simulink model "ards_model"  (R2020b)
settings: Solver=VariableStepAuto  StartTime=0.0  StopTime=480  MaxStep=0.2  RelTol=1e-3
model workspace: external: MAT-File model_workspace.mat (data not in the file)
values from neighbouring files (symbols this model uses):
  C_a_CO2_0 = 0.54    [model_workspace.mat]
  C_a_O2_0 = 0.1974    [model_workspace.mat]
  C_v_CO2_0 = 0.72    [model_workspace.mat]
  C_v_O2_0 = 0.13    [model_workspace.mat]
  moving_average_period = 5    [model_workspace.mat]
  P_ap_0 = 15    [model_workspace.mat]
  P_as_0 = 105.55    [model_workspace.mat]
  P_default = [105.55 4 15 6]    [model_workspace.mat]
  P_vs_0 = 4    [model_workspace.mat]
  Q_0 = 4.8    [model_workspace.mat]
undefined symbols (not defined in the file or in its folder): cRS, Pinsp, VT
libraries: pid_lib x1
(part 2 of 3)

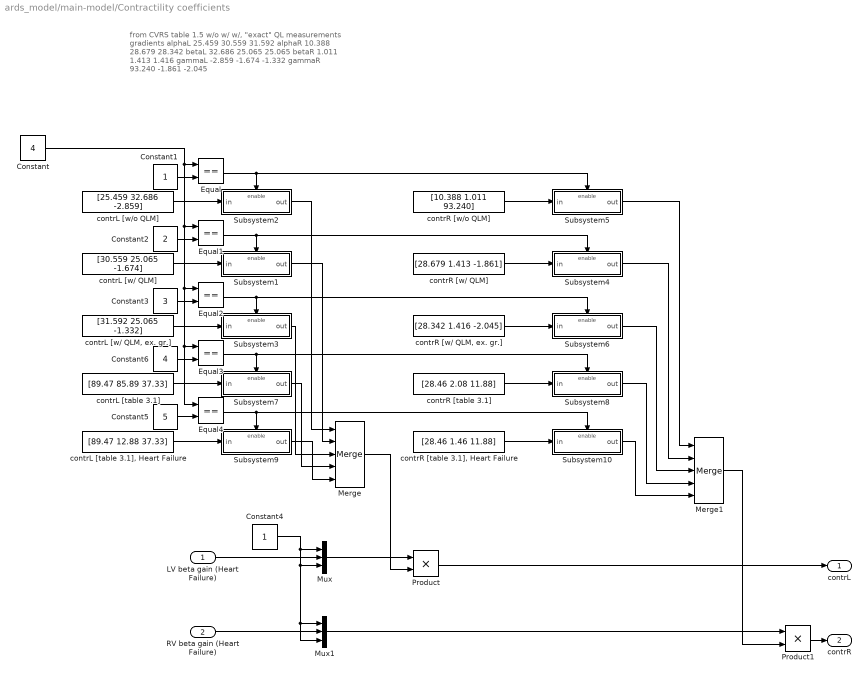
== system ards_model/main-model/Contractility coefficients ==
  note: from CVRS table 1.5
      | w/o w/ w/, "exact"
      | QL measurements gradients
      |
      | alphaL 25.459 30.559 31.592
      | alphaR 10.388 28.679 28.342
      | betaL 32.686 25.065 25.065
      | betaR 1.011 1.413 1.416
      | gammaL -2.859 -1.674 -1.332
      | gammaR 93.240 -1.861 -2.045
  LV beta gain (Heart Failure) : Inport
  RV beta gain (Heart Failure) : Inport  Port=2
  Constant : Constant  Value=4
  Constant1 : Constant
  Constant2 : Constant  Value=2
  Constant3 : Constant  Value=3
  Constant4 : Constant
  Constant5 : Constant  Value=5
  Constant6 : Constant  Value=4
  Equal{,1..4} (5 alike) : RelationalOperator  Operator===  OutDataTypeStr=boolean  RndMeth=Simplest
  Merge : Merge  Inputs=5
  Merge1 : Merge  Inputs=5
  Mux : Mux  Inputs=3
  Mux1 : Mux  Inputs=3
  Product : Product
  Product1 : Product
  Subsystem1 : Subsystem
  Subsystem10 : Subsystem
  Subsystem2 : Subsystem
  Subsystem3 : Subsystem
  Subsystem4 : Subsystem
  Subsystem5 : Subsystem
  Subsystem6 : Subsystem
  Subsystem7 : Subsystem
  Subsystem8 : Subsystem
  Subsystem9 : Subsystem
  contrL [table 3.1] : Constant  Value=[89.47 85.89 37.33]
  "contrL [table 3.1], Heart Failure" : Constant  Value=[89.47 12.88 37.33]
  "contrL [w/ QLM, ex. gr.]" : Constant  Value=[31.592 25.065 -1.332]
  contrL [w/ QLM] : Constant  Value=[30.559 25.065 -1.674]
  contrL [w/o QLM] : Constant  Value=[25.459 32.686 -2.859]
  contrR [table 3.1] : Constant  Value=[28.46 2.08 11.88]
  "contrR [table 3.1], Heart Failure" : Constant  Value=[28.46 1.46 11.88]
  "contrR [w/ QLM, ex. gr.]" : Constant  Value=[28.342 1.416 -2.045]
  contrR [w/ QLM] : Constant  Value=[28.679 1.413 -1.861]
  contrR [w/o QLM] : Constant  Value=[10.388 1.011 93.240]
  contrL : Outport  OutDataTypeStr=double  PortDimensions=3
  contrR : Outport  Port=2  OutDataTypeStr=double  PortDimensions=3
  wires:
  LV beta gain (Heart Failure)/1 -> Mux/2
  RV beta gain (Heart Failure)/1 -> Mux1/2
  Constant/1 -> Equal4/1, Equal3/1, Equal2/1, Equal1/1, Equal/1
  Constant1/1 -> Equal/2
  contrL [w/o QLM]/1 -> Subsystem2/1(in)
  contrL [w/ QLM]/1 -> Subsystem1/1(in)
  "contrL [w/ QLM, ex. gr.]"/1 -> Subsystem3/1(in)
  Equal/1 -> Subsystem5/Enable, Subsystem2/Enable
  Equal1/1 -> Subsystem4/Enable, Subsystem1/Enable
  Constant2/1 -> Equal1/2
  Equal2/1 -> Subsystem6/Enable, Subsystem3/Enable
  Constant3/1 -> Equal2/2
  Subsystem1/1(out) -> Merge/2
  Subsystem2/1(out) -> Merge/1
  Subsystem3/1(out) -> Merge/3
  contrR [w/o QLM]/1 -> Subsystem5/1(in)
  contrR [w/ QLM]/1 -> Subsystem4/1(in)
  "contrR [w/ QLM, ex. gr.]"/1 -> Subsystem6/1(in)
  Subsystem5/1(out) -> Merge1/1
  Subsystem4/1(out) -> Merge1/2
  Subsystem6/1(out) -> Merge1/3
  Constant4/1 -> Mux1/1, Mux1/3, Mux/3, Mux/1
  Mux/1 -> Product/1
  Merge/1 -> Product/2
  Mux1/1 -> Product1/1
  Merge1/1 -> Product1/2
  Product/1 -> contrL/1
  Product1/1 -> contrR/1
  contrL [table 3.1]/1 -> Subsystem7/1(in)
  Constant6/1 -> Equal3/2
  Equal3/1 -> Subsystem8/Enable, Subsystem7/Enable
  Subsystem7/1(out) -> Merge/4
  Subsystem8/1(out) -> Merge1/4
  contrR [table 3.1]/1 -> Subsystem8/1(in)
  "contrR [table 3.1], Heart Failure"/1 -> Subsystem10/1(in)
  Subsystem10/1(out) -> Merge1/5
  Subsystem9/1(out) -> Merge/5
  Equal4/1 -> Subsystem9/Enable, Subsystem10/Enable
  Constant5/1 -> Equal4/2
  "contrL [table 3.1], Heart Failure"/1 -> Subsystem9/1(in)

== system ards_model/main-model/Deadspace by PBW ==
  Weight : Inport  Unit=kg
  Constant1 : Constant  Value=0.0026
  Product2 : Product
  VD : Outport  Unit=L
  wires:
  Constant1/1 -> Product2/2
  Product2/1 -> VD/1  "VD"
  Weight/1 -> Product2/1  "PBW"

== system ards_model/main-model/Initial contractility ==
  H0 : Inport  Unit=1/min
  In3 : Inport  Port=2  OutDataTypeStr=double  PortDimensions=3
  In2 : Inport  Port=3  OutDataTypeStr=double  PortDimensions=3
  Demux : Demux  Outputs=2
  Demux1 : Demux  Outputs=2
  Product : Product  Inputs=*/*
  Product1 : Product  Inputs=*/*
  Selector : Selector  InputPortWidth=3  IndexOptions=Index vector (dialog)  Indices=[1 2]  OutputSizes=1
  Selector1 : Selector  InputPortWidth=3  IndexOptions=Index vector (dialog)  Indices=[1 2]  OutputSizes=1
  SL;0 : Outport  Unit=mmHg
  SR;0 : Outport  Port=2  Unit=mmHg
  wires:
  Product1/1 -> SL;0/1  "SL;0"
  Demux1/2 -> Product/3  "betaR"
  Product/1 -> SR;0/1  "SR;0"
  Demux1/1 -> Product/2  "alphaR"
  Selector/1 -> Demux/1
  Demux/1 -> Product1/2  "alphaL"
  H0/1 -> Product1/1, Product/1  "H0"
  In3/1 -> Selector/1  "contrL"
  Demux/2 -> Product1/3  "betaL"
  In2/1 -> Selector1/1  "contrR"
  Selector1/1 -> Demux1/1

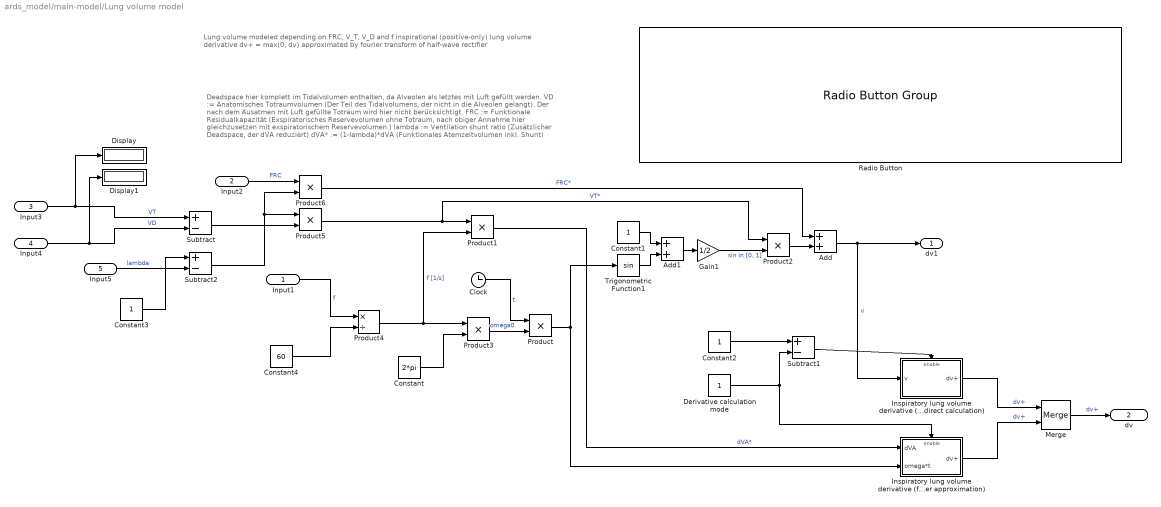
== system ards_model/main-model/Lung volume model ==
  note: Deadspace hier komplett im Tidalvolumen enthalten, da Alveolen als letztes mit Luft gefüllt werden.
      |
      | VD := Anatomisches Totraumvolumen (Der Teil des Tidalvolumens, der nicht in die Alveolen gelangt).
      | 	Der nach dem Ausatmen mit Luft gefüllte Totraum wird hier nicht berücksichtigt.
      | FRC := Funktionale Residualkapazität (Exspiratorisches Reservevolumen ohne Totraum,
      | 	nach obiger Annahme hier gleichzusetzen mit exspiratorischem Reservevolumen.)
      | lambda := Ventilation shunt ratio (Zusätzlicher Deadspace, der dVA reduziert)
      | dVA* := (1-lambda)*dVA (Funktionales Atemzeitvolumen inkl. Shunt)
  note: Lung volume modeled depending on FRC, V_T, V_D and f
      |
      | inspirational (positive-only) lung volume derivative dv+ = max(0, dv) approximated by fourier transform of half-wave rectifier
  Input1 : Inport  Unit=1/min
  Input2 : Inport  Port=2  Unit=L
  Input3 : Inport  Port=3  Unit=L
  Input4 : Inport  Port=4  Unit=L
  Input5 : Inport  Port=5  OutMin=0  OutMax=1  Unit=1
  Add : Sum
  Add1 : Sum
  Clock : Clock
  Constant : Constant  Value=2*pi
  Constant1 : Constant
  Constant2 : Constant
  Constant3 : Constant
  Constant4 : Constant  Value=60
  Derivative calculation mode : Constant
  Display : Display
  Display1 : Display
  Gain1 : Gain  Gain=1/2
  Inspiratory lung volume derivative (direct calculation) : Subsystem
  Inspiratory lung volume derivative (fourier approximation) : Subsystem
  Merge : Merge
  Product{,1..3,5..6} (6 alike) : Product
  Product4 : Product  Inputs=*/
  Radio Button : RadioButtonGroup  SelectedLabel=Fourier approximation (continuous)  ButtonGroupName=Select mode
      settings: Values={{'Direct calculation (with discontinuities)', 'Fourier approximation (continuous)'}, [0 1]}
  Subtract : Sum  Inputs=+-
  Subtract1 : Sum  Inputs=+-
  Subtract2 : Sum  Inputs=+-
  Trigonometric Function1 : Trigonometry
  dv1 : Outport  Unit=L
  dv : Outport  Port=2  Unit=L/s
  wires:
  Product3/1 -> Product/2  "omega0"
  Product4/1 -> Product3/1, Product1/2  "f [1/s]"
  Clock/1 -> Product/1  "t"
  Trigonometric Function1/1 -> Add1/2
  Product2/1 -> Add/2
  Product6/1 -> Add/1  "FRC*"
  Add/1 -> Inspiratory lung volume derivative (direct calculation)/1(v), dv1/1  "v"
  Add1/1 -> Gain1/1
  Constant1/1 -> Add1/1
  Input3/1 -> Display/1, Subtract/1  "VT"
  Input4/1 -> Subtract/2, Display1/1  "VD"
  Constant/1 -> Product3/2
  Product/1 -> Inspiratory lung volume derivative (fourier approximation)/2(omega*t), Trigonometric Function1/1
  Constant4/1 -> Product4/2
  Input1/1 -> Product4/1  "f"
  Gain1/1 -> Product2/2  "sin in [0, 1]"
  Product5/1 -> Product1/1, Product2/1  "VT*"
  Product1/1 -> Inspiratory lung volume derivative (fourier approximation)/1(dVA)  "dVA*"
  Inspiratory lung volume derivative (fourier approximation)/1(dv+) -> Merge/2  "dv+"
  Constant2/1 -> Subtract1/1
  Derivative calculation mode/1 -> Subtract1/2, Inspiratory lung volume derivative (fourier approximation)/Enable
  Inspiratory lung volume derivative (direct calculation)/1(dv+) -> Merge/1  "dv+"
  Merge/1 -> dv/1  "dv+"
  Subtract1/1 -> Inspiratory lung volume derivative (direct calculation)/Enable
  Input5/1 -> Subtract2/2  "lambda"
  Constant3/1 -> Subtract2/1
  Subtract/1 -> Product5/2
  Subtract2/1 -> Product6/2, Product5/1
  Input2/1 -> Product6/1  "FRC"

== system ards_model/main-model/Metabolic Parameters ==
  note: S_T = 50 lit (Fincham-Tehrani)
      | S_T = 13 lit (Tehrani DSS)
  Equivalent gas storage (body tissue) [lit] : Constant  Value=13
  Equivalent gas storage (body tissue) [lit]1 : Constant  Value=50
  Equivalent gas storage (brain) [lit] : Constant  Value=1.1
  "Metabolic rate (CO2, body tissue) [lit/s]" : Constant  Value=0.00287
  "Metabolic rate (CO2, brain) [lit/s]" : Constant  Value=0.0009
  "Metabolic rate (O2, body tissue, positive) [lit/s]" : Constant  Value=0.00352
  "Metabolic rate (O2, brain, positive) [lit/s]" : Constant  Value=0.000925
  Multiply : Gain  Gain=-1
  Multiply1 : Gain  Gain=-1
  Mux : Mux  Inputs=3
  Mux1 : Mux  Inputs=3
  Output : Outport  PortDimensions=3
  Output1 : Outport  Port=2  PortDimensions=3
  wires:
  Equivalent gas storage (body tissue) [lit]1/1 -> Mux/1  "S_T"
  "Metabolic rate (O2, body tissue, positive) [lit/s]"/1 -> Multiply1/1  "-MRT;O2"
  "Metabolic rate (O2, brain, positive) [lit/s]"/1 -> Multiply/1  "-MRB;O2"
  "Metabolic rate (CO2, body tissue) [lit/s]"/1 -> Mux/3  "MRT;CO2"
  Multiply1/1 -> Mux/2  "MRT;O2"
  Multiply/1 -> Mux1/2  "MRB;O2"
  Equivalent gas storage (brain) [lit]/1 -> Mux1/1  "S_B"
  "Metabolic rate (CO2, brain) [lit/s]"/1 -> Mux1/3  "MRB;CO2"
  Mux/1 -> Output/1  "paramsT"
  Mux1/1 -> Output1/1  "paramsB"

== system ards_model/main-model/Predicted Body Weight ==
  note: Predicted body weight
      | Source: Ventilation with lower tidal volumes [...], page 3
  height : Inport  Unit=m
  Input : Inport  Port=2  OutDataTypeStr=boolean
  Add4 : Sum  Inputs=+-
  Constant1 : Constant  Value=1.524
  Constant3 : Constant  Value=0
  Gain : Gain  Gain=91
  IfThenElse : Subsystem
  Max : MinMax  Function=max  Inputs=2
  Subtract1 : Sum
  female : Constant  Value=45.5
  male : Constant  Value=50
  Weight : Outport  Unit=kg
  wires:
  Max/1 -> Gain/1
  Constant1/1 -> Add4/2
  Gain/1 -> Subtract1/1
  Constant3/1 -> Max/2
  height/1 -> Add4/1  "height"
  Subtract1/1 -> Weight/1  "PBW"
  Add4/1 -> Max/1
  female/1 -> IfThenElse/2(then)
  male/1 -> IfThenElse/3(else)
  IfThenElse/1(out) -> Subtract1/2
  Input/1 -> IfThenElse/1(if)  "female"

== system ards_model/main-model/Tissue-Brain fork ratio ==
  note: Tissue-Brain fork ratio
      | Use blood flow rates from [TehraniAbbasi] to calculate fork ratio
  Add : Sum
  Blood flow in body tissue [lit/s] : Constant  Value=0.07083
  Blood flow in brain [lit/s] : Constant  Value=0.0125
  Divide : Product  Inputs=*/
  QT/Qco : Outport  Unit=1
  wires:
  Divide/1 -> QT/Qco/1  "QT/Qs"
  Add/1 -> Divide/2  "qs"
  Blood flow in brain [lit/s]/1 -> Add/2  "qB"
  Blood flow in body tissue [lit/s]/1 -> Divide/1, Add/1  "qT"

== system ards_model/main-model/Total metabolic rate ==
  MRT;O2 : Inport  Unit=L/s
  MRB;O2 : Inport  Port=2  Unit=L/s
  Add : Sum  Inputs=--
  Constant : Constant  Value=60
  Product : Product
  MR_;O2 : Outport  Unit=L/min
  wires:
  Product/1 -> MR_;O2/1  "-MR_;O2"
  Constant/1 -> Product/2
  MRB;O2/1 -> Add/2
  Add/1 -> Product/1
  MRT;O2/1 -> Add/1

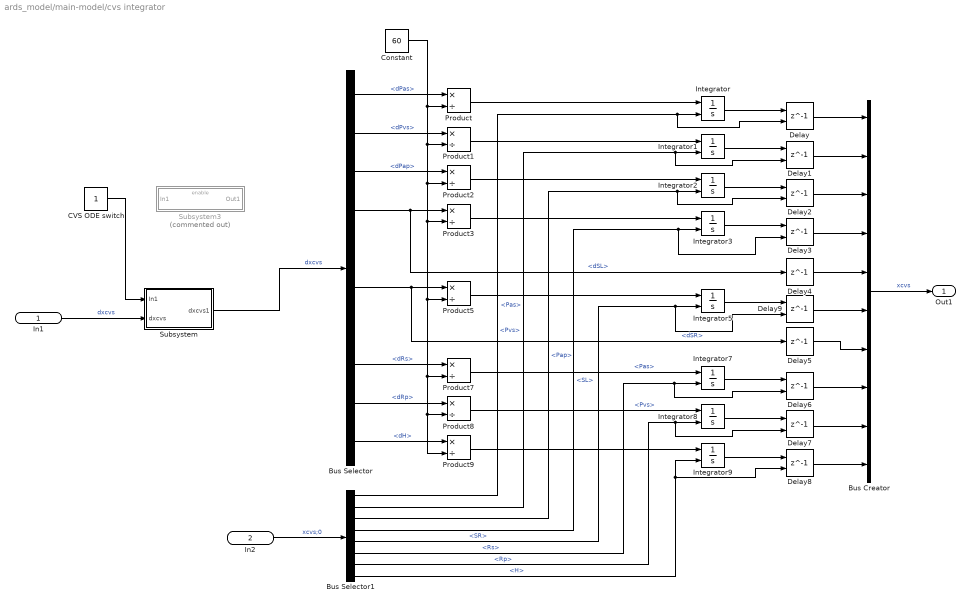
== system ards_model/main-model/cvs integrator ==
  In1 : Inport  OutDataTypeStr=Bus: CardioVascularStateDerivative
  In2 : Inport  Port=2  OutDataTypeStr=Bus: CardioVascularState
  Bus Creator : BusCreator  Inputs=10  OutDataTypeStr=Bus: CardioVascularState
      settings: InheritFromInputs=off
  Bus Selector : BusSelector  OutputSignals=dPas,dPvs,dPap,dSL,dsigmaL,dSR,dsigmaR,dRs,dRp,dH
  Bus Selector1 : BusSelector  OutputSignals=Pas,Pvs,Pap,SL,SR,Rs,Rp,H
  CVS ODE switch : Constant
  Constant : Constant  Value=60
  Delay{,1..3,6..9} (8 alike) : Delay  DelayLength=1  InitialConditionSource=Input port
      settings: InputPortMap=u0,p4
  Delay4 : Delay  DelayLength=1
  Delay5 : Delay  DelayLength=1
  Integrator{,1..3,5,7..9} (8 alike) : Integrator  InitialConditionSource=external
  Product{,1..3,5,7..9} (8 alike) : Product  Inputs=*/
  Subsystem : Subsystem
  Subsystem3 : Subsystem  Commented=on
  Out1 : Outport  OutDataTypeStr=Bus: CardioVascularState
  wires:
  In2/1 -> Bus Selector1/1  "xcvs;0"
  Bus Creator/1 -> Out1/1  "xcvs"
  Bus Selector/1 -> Product/1  "<dPas>"
  Constant/1 -> Product9/2, Product8/2, Product7/2, Product5/2, Product3/2, Product2/2, Product1/2, Product/2
  Product/1 -> Integrator/1
  Product1/1 -> Integrator1/1
  Product2/1 -> Integrator2/1
  Bus Selector/3 -> Product2/1  "<dPap>"
  Bus Selector/2 -> Product1/1  "<dPvs>"
  Product3/1 -> Integrator3/1
  Bus Selector/4 -> Delay4/1, Product3/1  "<dSL>"
  Product9/1 -> Integrator9/1
  Product5/1 -> Integrator5/1
  Bus Selector/6 -> Delay5/1, Product5/1  "<dSR>"
  Bus Selector/8 -> Product7/1  "<dRs>"
  Bus Selector/9 -> Product8/1  "<dRp>"
  Bus Selector/10 -> Product9/1  "<dH>"
  Bus Selector1/1 -> Delay/2, Integrator/2  "<Pas>"
  Bus Selector1/2 -> Delay1/2, Integrator1/2  "<Pvs>"
  Bus Selector1/3 -> Delay2/2, Integrator2/2  "<Pap>"
  Bus Selector1/4 -> Delay3/2, Integrator3/2  "<SL>"
  Bus Selector1/5 -> Delay9/2, Integrator5/2  "<SR>"
  Bus Selector1/6 -> Delay6/2, Integrator7/2  "<Rs>"
  Bus Selector1/7 -> Delay7/2, Integrator8/2  "<Rp>"
  Integrator/1 -> Delay/1
  Integrator1/1 -> Delay1/1
  Integrator2/1 -> Delay2/1
  Integrator3/1 -> Delay3/1
  Delay5/1 -> Bus Creator/7
  Integrator9/1 -> Delay8/1
  Integrator8/1 -> Delay7/1
  Integrator7/1 -> Delay6/1
  Product8/1 -> Integrator8/1  "<Pvs>"
  Product7/1 -> Integrator7/1  "<Pas>"
  Bus Selector1/8 -> Delay8/2, Integrator9/2  "<H>"
  Delay4/1 -> Bus Creator/5
  Delay3/1 -> Bus Creator/4
  Delay2/1 -> Bus Creator/3
  Delay1/1 -> Bus Creator/2
  Delay/1 -> Bus Creator/1
  Delay6/1 -> Bus Creator/8
  Delay7/1 -> Bus Creator/9
  Delay8/1 -> Bus Creator/10
  Integrator5/1 -> Delay9/1
  Delay9/1 -> Bus Creator/6
  Subsystem/1(dxcvs1) -> Bus Selector/1  "dxcvs"
  In1/1 -> Subsystem/2(dxcvs)  "dxcvs"
  CVS ODE switch/1 -> Subsystem/1(In1)

== system ards_model/main-model/cvs_bkst ==
  Input : Inport  OutDataTypeStr=Bus: CardioVascularState
  Input2 : Inport  Port=2  OutDataTypeStr=Bus: CardioVascularState
  Input1 : Inport  Port=3  OutDataTypeStr=Bus: RespiratoryStateExtended
  body surface : Inport  Port=4  Unit=m^2
  CvO1 : Inport  Port=5  Unit=L/min
  Input4 : Inport  Port=6  OutDataTypeStr=double  PortDimensions=3
  Input5 : Inport  Port=7  OutDataTypeStr=double  PortDimensions=3
  Input3 : InportShadow  OutDataTypeStr=Bus: CardioVascularState
  ODEs : Subsystem
  Subsystem : Subsystem
  calculations : Subsystem  ReferencedSubsystem=cvs_calculations
  initial calculations : Subsystem  Commented=on  ReferencedSubsystem=cvs_calculations
  Output : Outport  OutDataTypeStr=Bus: CardioVascularStateDerivative
  Output1 : Outport  Port=2  OutDataTypeStr=Bus: CardioVascularStateExtended
  wires:
  Input/1 -> calculations/1  "xcvs"
  body surface/1 -> initial calculations/2, calculations/2  "surface"
  Input4/1 -> ODEs/3(Input4)  "contrL"
  Input5/1 -> ODEs/4(Input5)  "contrR"
  Input3/1 -> ODEs/5(Input)  "xcvs"
  Input1/1 -> ODEs/6(Input1)  "xrsExt"
  CvO1/1 -> ODEs/7(CvO1)  "-MR_;O2"
  Input2/1 -> initial calculations/1  "xcvs;0"
  calculations/1 -> Subsystem/1(In1)  "xcvsExt"
  ODEs/1(dxcvs [/min]) -> Output/1  "dxcvs"
  calculations/2 -> ODEs/2(c_)
  Subsystem/1(Out1) -> Output1/1, ODEs/1(xcvsExt)

== system ards_model/main-model/rs integrator ==
  In1 : Inport  OutDataTypeStr=Bus: RespiratoryStateDerivative
  In2 : Inport  Port=2  OutDataTypeStr=Bus: RespiratoryState
  Bus Creator1 : BusCreator  Inputs=6  OutDataTypeStr=Bus: RespiratoryState
      settings: InheritFromInputs=off
  Bus Selector1 : BusSelector  OutputSignals=dPaxO2,dPaxCO2,dCvBO2,dCvBCO2,dCvTO2,dCvTCO2
  Bus Selector2 : BusSelector  OutputSignals=PaxO2,PaxCO2,CvBO2,CvBCO2,CvTO2,CvTCO2
  Delay{,1..5} (6 alike) : Delay  DelayLength=1  InitialConditionSource=Input port
      settings: InputPortMap=u0,p4
  Integrator{,1..5} (6 alike) : Integrator  InitialConditionSource=external
  RS ODE switch : Constant
  Subsystem : Subsystem
  Out1 : Outport  OutDataTypeStr=Bus: RespiratoryState
  wires:
  Integrator/1 -> Delay/1
  Bus Selector2/3 -> Integrator2/2, Delay2/2  "<CvBO2>"
  Bus Selector2/6 -> Delay5/2, Integrator5/2  "<CvTCO2>"
  Bus Selector2/1 -> Delay/2, Integrator/2  "<PaxO2>"
  Bus Selector2/2 -> Delay1/2, Integrator1/2  "<PaxCO2>"
  Integrator4/1 -> Delay4/1
  Integrator2/1 -> Delay2/1
  Bus Selector1/4 -> Integrator3/1  "<dCvBCO2>"
  Integrator1/1 -> Delay1/1
  Integrator5/1 -> Delay5/1
  Bus Selector1/3 -> Integrator2/1  "<dCvBO2>"
  Bus Selector2/4 -> Delay3/2, Integrator3/2  "<CvBCO2>"
  Delay1/1 -> Bus Creator1/2
  Bus Selector1/5 -> Integrator4/1  "<dCvTO2>"
  Delay4/1 -> Bus Creator1/5
  Delay2/1 -> Bus Creator1/3
  Bus Selector2/5 -> Delay4/2, Integrator4/2  "<CvTO2>"
  Delay5/1 -> Bus Creator1/6
  Integrator3/1 -> Delay3/1
  Delay3/1 -> Bus Creator1/4
  Delay/1 -> Bus Creator1/1
  Bus Selector1/1 -> Integrator/1  "<dPaxO2>"
  Bus Selector1/6 -> Integrator5/1  "<dCvTCO2>"
  Bus Selector1/2 -> Integrator1/1  "<dPaxCO2>"
  Bus Creator1/1 -> Out1/1  "xrs"
  In2/1 -> Bus Selector2/1  "xrs;0"
  Subsystem/1(dxcvs1) -> Bus Selector1/1  "dxrs"
  RS ODE switch/1 -> Subsystem/1(In1)
  In1/1 -> Subsystem/2(dxcvs)  "dxrs"

== system ards_model/main-model/rs_tehrani ==
  Qco7 : Inport  OutDataTypeStr=Bus: RespiratoryState  Unit=liter/minute
  Qco2 : Inport  Port=2  OutDataTypeStr=Bus: RespiratoryState  Unit=liter/minute
  Qco : Inport  Port=3  OutDataTypeStr=Bus: CardioVascularStateExtended  Unit=liter/minute
  v : Inport  Port=4  Unit=L
  dv+ : Inport  Port=5  Unit=liter/second
  Pamb* : Inport  Port=6  Unit=mmHg
  Fi;O2 : Inport  Port=7  Unit=1
  Fi;CO2 : Inport  Port=8  Unit=1
  rho : Inport  Port=9  Unit=1
  QT8 : Inport  Port=10  PortDimensions=3
  QT4 : Inport  Port=11  PortDimensions=3
  QT;0/Qco;0 : Inport  Port=12  Unit=1
  Fi;O1 : InportShadow  Port=7  Unit=1
  ODEs : Subsystem
  calculations : Subsystem  ReferencedSubsystem=tehrani_rs_calculations
  initial calculations : Subsystem  Commented=on  ReferencedSubsystem=tehrani_rs_calculations
  Output : Outport  OutDataTypeStr=Bus: RespiratoryStateDerivative
  Output1 : Outport  Port=2  OutDataTypeStr=Bus: RespiratoryStateExtended
  wires:
  Qco/1 -> initial calculations/2, calculations/2  "xcvsExt"
  Fi;O1/1 -> initial calculations/3, calculations/3  "Fi;O2"
  rho/1 -> initial calculations/4, calculations/4  "rho"
  QT;0/Qco;0/1 -> initial calculations/5, calculations/5  "QT/Qs"
  Qco7/1 -> calculations/1  "xrs"
  Qco2/1 -> initial calculations/1  "xrs0"
  Pamb*/1 -> ODEs/5(Pamb*)  "Pamb"
  v/1 -> ODEs/6(v)  "v"
  dv+/1 -> ODEs/7(dv+)  "dv+"
  Fi;O2/1 -> ODEs/8(Fi;O2)  "Fi;O2"
  Fi;CO2/1 -> ODEs/9(Fi;CO2)  "Fi;CO2"
  calculations/2 -> ODEs/2(inpp*)
  calculations/3 -> ODEs/3(inpB)
  calculations/4 -> ODEs/4(inpT)
  ODEs/1(dxrs) -> Output/1  "dxrs"
  QT8/1 -> ODEs/11(QT1)  "paramsT"
  QT4/1 -> ODEs/10(QT4)  "paramsB"
  calculations/1 -> Output1/1, ODEs/1(xrsExt)  "xrsExt"

== system ards_model/Predicted Body Weight/IfThenElse/Subsystem1 ==
  in : Inport
  Enable : EnablePort
  out : Outport
  wires:
  in/1 -> out/1

== system ards_model/Predicted Body Weight/IfThenElse/Subsystem2 ==
  in : Inport
  Enable : EnablePort
  out : Outport
  wires:
  in/1 -> out/1

== system ards_model/ards_classification/ARDS level score calculation/Subsystem ==
  in : Inport
  Enable : EnablePort
  out : Outport
  wires:
  in/1 -> out/1

== system ards_model/ards_classification/ARDS level score calculation/Subsystem1 ==
  in : Inport
  Enable : EnablePort
  out : Outport
  wires:
  in/1 -> out/1

== system ards_model/ards_classification/ARDS level score calculation/Subsystem2 ==
  in : Inport
  Enable : EnablePort
  out : Outport
  wires:
  in/1 -> out/1

== system ards_model/ards_classification/ARDS level score calculation/Subsystem3 ==
  in : Inport
  Enable : EnablePort
  out : Outport
  wires:
  in/1 -> out/1

== system ards_model/ards_classification/Berlin definition/PEEP bound ==
  PEEP : Inport  Unit=mbar
  Constant : Constant  Value=5
  GreaterThanOrEqual : RelationalOperator  OutDataTypeStr=boolean  RndMeth=Simplest
  Subsystem2 : Subsystem  ReferencedSubsystem=convert_mbar_to_cmh2o
  Out1 : Outport  OutDataTypeStr=boolean
  wires:
  Constant/1 -> GreaterThanOrEqual/2
  Subsystem2/1 -> GreaterThanOrEqual/1  "PEEP [cmH2O]"
  GreaterThanOrEqual/1 -> Out1/1  "ispeep"
  PEEP/1 -> Subsystem2/1

== system ards_model/ards_classification/Berlin definition/ards_level ==
  horowitz : Inport  Unit=mmHg
  Fi;O2 : Inport  Port=2  Unit=1
  altitude : Inport  Port=3  Unit=m
  Pamb : Inport  Port=4  Unit=mmHg
  Input : Inport  Port=5
  AND : Logic  IconShape=distinctive  AllPortsSameDT=off  OutDataTypeStr=boolean
  AND1 : Logic  IconShape=distinctive  AllPortsSameDT=off  OutDataTypeStr=boolean
  AND2 : Logic  IconShape=distinctive  AllPortsSameDT=off  OutDataTypeStr=boolean
  NOT : Logic  Operator=NOT  IconShape=distinctive  AllPortsSameDT=off  OutDataTypeStr=boolean
  NOT1 : Logic  Operator=NOT  IconShape=distinctive  AllPortsSameDT=off  OutDataTypeStr=boolean
  OR : Logic  Operator=OR  IconShape=distinctive  AllPortsSameDT=off  OutDataTypeStr=boolean
  ards_level_string : Subsystem
  ards_level_switch : Subsystem
  Out1 : Outport
  ards : Outport  Port=2
  no : Outport  Port=3
  mild : Outport  Port=4
  moderate : Outport  Port=5
  severe : Outport  Port=6
  wires:
  AND/1 -> ards_level_string/1(In1), severe/1  "severe"
  AND2/1 -> ards_level_string/3(In3), mild/1  "mild"
  AND1/1 -> ards_level_string/2(In2), moderate/1  "moderate"
  horowitz/1 -> ards_level_switch/1(horowitz)
  Pamb/1 -> ards_level_switch/4(Pamb)
  ards_level_string/1(ards_level) -> Out1/1  "level_string"
  NOT/1 -> ards/1  "ards"
  Input/1 -> AND2/2, AND1/2, AND/2, NOT1/1  "ispeep"
  ards_level_switch/1(issevere) -> AND/1  "severe"
  ards_level_switch/2(ismoderate) -> AND1/1  "moderate"
  ards_level_switch/3(ismild) -> AND2/1  "mild"
  OR/1 -> ards_level_string/4(In4), NOT/1, no/1  "no"
  ards_level_switch/4(isno) -> OR/1  "no"
  NOT1/1 -> OR/2
  altitude/1 -> ards_level_switch/3(Pamb1)
  Fi;O2/1 -> ards_level_switch/2(horowitz1)

== system ards_model/ards_classification/LVEF_score/Enabled Subsystem ==
  In1 : Inport
  Enable : EnablePort
  Out1 : Outport
  wires:
  In1/1 -> Out1/1

== system ards_model/ards_classification/LVEF_score/Enabled Subsystem1 ==
  In1 : Inport
  Enable : EnablePort
  Out1 : Outport
  wires:
  In1/1 -> Out1/1

== system ards_model/ards_classification/LVEF_score/Enabled Subsystem2 ==
  In1 : Inport
  Enable : EnablePort
  Out1 : Outport
  wires:
  In1/1 -> Out1/1

== system ards_model/ards_classification/NTproBNP_score/Enabled Subsystem ==
  In1 : Inport
  Enable : EnablePort
  Out1 : Outport
  wires:
  In1/1 -> Out1/1

== system ards_model/ards_classification/NTproBNP_score/Enabled Subsystem1 ==
  In1 : Inport
  Enable : EnablePort
  Out1 : Outport
  wires:
  In1/1 -> Out1/1

== system ards_model/ards_classification/NTproBNP_score/Enabled Subsystem2 ==
  In1 : Inport
  Enable : EnablePort
  Out1 : Outport
  wires:
  In1/1 -> Out1/1

== system ards_model/ards_classification/RHF_risk_level_string/Subsystem ==
  in : Inport
  Enable : EnablePort
  out : Outport
  wires:
  in/1 -> out/1

== system ards_model/ards_classification/RHF_risk_level_string/Subsystem1 ==
  in : Inport
  Enable : EnablePort
  out : Outport
  wires:
  in/1 -> out/1

== system ards_model/ards_classification/RHF_risk_level_string/Subsystem2 ==
  in : Inport
  Enable : EnablePort
  out : Outport
  wires:
  in/1 -> out/1

== system ards_model/ards_classification/RHF_risk_level_string/Subsystem3 ==
  in : Inport
  Enable : EnablePort
  out : Outport
  wires:
  in/1 -> out/1

== system ards_model/ards_classification/eGFR_CKD-EPI/alpha ==
  In1 : Inport
  Constant : Constant
  Enabled Subsystem : Subsystem  TreatAsAtomicUnit=on
  Enabled Subsystem1 : Subsystem  TreatAsAtomicUnit=on
  Equal : RelationalOperator  Operator===  OutDataTypeStr=boolean  RndMeth=Simplest
  Merge : Merge
  NOT : Logic  Operator=NOT  IconShape=distinctive  AllPortsSameDT=off  OutDataTypeStr=boolean
  alphaM : Constant  Value=-0.411
  alphaW : Constant  Value=-0.329
  Out1 : Outport
  wires:
  Merge/1 -> Out1/1
  Enabled Subsystem/1(Out1) -> Merge/1
  NOT/1 -> Enabled Subsystem1/Enable
  alphaM/1 -> Enabled Subsystem1/1(In1)
  alphaW/1 -> Enabled Subsystem/1(In1)
  In1/1 -> Enabled Subsystem/Enable, NOT/1
  Enabled Subsystem1/1(Out1) -> Merge/2
  Constant/1 -> Equal/1

== system ards_model/ards_classification/eGFR_CKD-EPI/kappa ==
  In1 : Inport
  Constant : Constant
  Enabled Subsystem : Subsystem  TreatAsAtomicUnit=on
  Enabled Subsystem1 : Subsystem  TreatAsAtomicUnit=on
  Equal : RelationalOperator  Operator===  OutDataTypeStr=boolean  RndMeth=Simplest
  Merge : Merge
  NOT : Logic  Operator=NOT  IconShape=distinctive  AllPortsSameDT=off  OutDataTypeStr=boolean
  kappaM : Constant  Value=0.9
  kappaW : Constant  Value=0.7
  Out1 : Outport
  wires:
  Enabled Subsystem1/1(Out1) -> Merge/2
  In1/1 -> Enabled Subsystem/Enable, NOT/1
  kappaW/1 -> Enabled Subsystem/1(In1)
  kappaM/1 -> Enabled Subsystem1/1(In1)
  NOT/1 -> Enabled Subsystem1/Enable
  Enabled Subsystem/1(Out1) -> Merge/1
  Merge/1 -> Out1/1
  Constant/1 -> Equal/1

== system ards_model/ards_classification/eGFR_CKD-EPI/sex factor ==
  In1 : Inport
  Constant : Constant
  Enabled Subsystem : Subsystem  TreatAsAtomicUnit=on
  Enabled Subsystem1 : Subsystem  TreatAsAtomicUnit=on
  Equal : RelationalOperator  Operator===  OutDataTypeStr=boolean  RndMeth=Simplest
  M : Constant
  Merge : Merge
  NOT : Logic  Operator=NOT  IconShape=distinctive  AllPortsSameDT=off  OutDataTypeStr=boolean
  W : Constant  Value=1.018
  Out1 : Outport
  wires:
  Enabled Subsystem1/1(Out1) -> Merge/2
  In1/1 -> Enabled Subsystem/Enable, NOT/1
  W/1 -> Enabled Subsystem/1(In1)
  M/1 -> Enabled Subsystem1/1(In1)
  NOT/1 -> Enabled Subsystem1/Enable
  Enabled Subsystem/1(Out1) -> Merge/1
  Merge/1 -> Out1/1
  Constant/1 -> Equal/1

== system ards_model/ards_classification/eGFR_CKD-EPI/skin color factor ==
  In1 : Inport
  B : Constant  Value=1.159
  Constant : Constant
  Enabled Subsystem : Subsystem  TreatAsAtomicUnit=on
  Enabled Subsystem1 : Subsystem  TreatAsAtomicUnit=on
  Equal : RelationalOperator  Operator===  OutDataTypeStr=boolean  RndMeth=Simplest
  Merge : Merge
  NOT : Logic  Operator=NOT  IconShape=distinctive  AllPortsSameDT=off  OutDataTypeStr=boolean
  W : Constant
  Out1 : Outport
  wires:
  Merge/1 -> Out1/1
  Enabled Subsystem/1(Out1) -> Merge/1
  NOT/1 -> Enabled Subsystem1/Enable
  W/1 -> Enabled Subsystem1/1(In1)
  B/1 -> Enabled Subsystem/1(In1)
  In1/1 -> NOT/1, Enabled Subsystem/Enable
  Enabled Subsystem1/1(Out1) -> Merge/2
  Constant/1 -> Equal/1

== system ards_model/ards_classification/logFon_score/Compliance ==
  <height> : Inport  Unit=m
  <weight> : Inport  Port=2  Unit=kg
  Blood volume estimate : Subsystem  TreatAsAtomicUnit=on
  Body surface estimate : Subsystem  TreatAsAtomicUnit=on
  Initial blood volume distribution : Subsystem  TreatAsAtomicUnit=on
  Mux : Mux
  Selector : Selector  InputPortWidth=4  IndexOptions=Index vector (dialog)  Indices=[1]  OutputSizes=1
  Vessel compliances : Subsystem  TreatAsAtomicUnit=on
  cas : Outport  Unit=L/mmHg
  wires:
  Mux/1 -> Selector/1  "c_"
  Vessel compliances/1(cas) -> Mux/1  "cas"
  Vessel compliances/4(cvp) -> Mux/4  "cvp"
  Blood volume estimate/1(Vtot) -> Initial blood volume distribution/1(Vtot)  "Vtot"
  Initial blood volume distribution/4(V_as3) -> Vessel compliances/4(In8)  "Vvp;0"
  Vessel compliances/3(cap) -> Mux/3  "cap"
  Initial blood volume distribution/2(V_as1) -> Vessel compliances/2(In6)  "Vvs;0"
  Initial blood volume distribution/1(V_as) -> Vessel compliances/1(In5)  "Vas;0"
  Vessel compliances/2(cvs) -> Mux/2  "cvs"
  Body surface estimate/1(surface) -> Blood volume estimate/1(surface)  "surface"
  Initial blood volume distribution/3(V_as2) -> Vessel compliances/3(In7)  "Vap;0"
  <weight>/1 -> Body surface estimate/2(Weight)
  Selector/1 -> cas/1  "cas"
  <height>/1 -> Body surface estimate/1(height)

== system ards_model/ards_classification/logFon_score/peak Pas ==
  note: MAP = DBP + tau_syst * (SBP - DBP)
      | [Moran et al.: "Calculation of mean arterial pressure during exercise as a function of Heart Rate"]
  <Pas> : Inport
  <H> : Inport  Port=2
  <Vstr> : Inport  Port=3
  cas : Inport  Port=4
  Add : Sum
  Add1 : Sum
  Add2 : Sum  Inputs=+-
  Constant : Constant  Value=40
  Constant1 : Constant
  Divide : Product  Inputs=*/
  Divide1 : Product  Inputs=*/
  Duration of heart cycle : Subsystem  TreatAsAtomicUnit=on  ReferencedSubsystem=cvrs_heart_cycle
  Max : MinMax  Function=max  Inputs=2
  Product : Product
  Product1 : Product
  Subtract : Sum  Inputs=+-
  Pas;diast : Outport
  Pas;syst : Outport  Port=2
  wires:
  Add/1 -> Divide1/2
  Product/1 -> Add1/2
  Constant1/1 -> Subtract/1
  Duration of heart cycle/2 -> Add/2, Divide1/1  "tsyst"
  Divide/1 -> Product1/2, Product/2  "deltaPas"
  Duration of heart cycle/1 -> Add/1  "tdiast"
  Subtract/1 -> Product/1  "taudiast"
  cas/1 -> Divide/2
  Divide1/1 -> Product1/1, Subtract/2  "tausyst"
  <Vstr>/1 -> Divide/1
  Add1/1 -> Pas;syst/1  "Pas;syst"
  <Pas>/1 -> Add2/1, Add1/1
  Max/1 -> Duration of heart cycle/1
  Constant/1 -> Max/2
  <H>/1 -> Max/1
  Product1/1 -> Add2/2
  Add2/1 -> Pas;diast/1  "Pas;diast"

== system ards_model/main-model/Contractility coefficients/Subsystem1 ==
  in : Inport  OutDataTypeStr=double  PortDimensions=3
  Enable : EnablePort
  out : Outport  OutDataTypeStr=double  PortDimensions=3
  wires:
  in/1 -> out/1

== system ards_model/main-model/Contractility coefficients/Subsystem10 ==
  in : Inport  OutDataTypeStr=double  PortDimensions=3
  Enable : EnablePort
  out : Outport  OutDataTypeStr=double  PortDimensions=3
  wires:
  in/1 -> out/1

== system ards_model/main-model/Contractility coefficients/Subsystem2 ==
  in : Inport  OutDataTypeStr=double  PortDimensions=3
  Enable : EnablePort
  out : Outport  OutDataTypeStr=double  PortDimensions=3
  wires:
  in/1 -> out/1

== system ards_model/main-model/Contractility coefficients/Subsystem3 ==
  in : Inport  OutDataTypeStr=double  PortDimensions=3
  Enable : EnablePort
  out : Outport  OutDataTypeStr=double  PortDimensions=3
  wires:
  in/1 -> out/1

== system ards_model/main-model/Contractility coefficients/Subsystem4 ==
  in : Inport  OutDataTypeStr=double  PortDimensions=3
  Enable : EnablePort
  out : Outport  OutDataTypeStr=double  PortDimensions=3
  wires:
  in/1 -> out/1

== system ards_model/main-model/Contractility coefficients/Subsystem5 ==
  in : Inport  OutDataTypeStr=double  PortDimensions=3
  Enable : EnablePort
  out : Outport  OutDataTypeStr=double  PortDimensions=3
  wires:
  in/1 -> out/1

== system ards_model/main-model/Contractility coefficients/Subsystem6 ==
  in : Inport  OutDataTypeStr=double  PortDimensions=3
  Enable : EnablePort
  out : Outport  OutDataTypeStr=double  PortDimensions=3
  wires:
  in/1 -> out/1

== system ards_model/main-model/Contractility coefficients/Subsystem7 ==
  in : Inport  OutDataTypeStr=double  PortDimensions=3
  Enable : EnablePort
  out : Outport  OutDataTypeStr=double  PortDimensions=3
  wires:
  in/1 -> out/1

== system ards_model/main-model/Contractility coefficients/Subsystem8 ==
  in : Inport  OutDataTypeStr=double  PortDimensions=3
  Enable : EnablePort
  out : Outport  OutDataTypeStr=double  PortDimensions=3
  wires:
  in/1 -> out/1

== system ards_model/main-model/Contractility coefficients/Subsystem9 ==
  in : Inport  OutDataTypeStr=double  PortDimensions=3
  Enable : EnablePort
  out : Outport  OutDataTypeStr=double  PortDimensions=3
  wires:
  in/1 -> out/1

== system ards_model/main-model/Lung volume model/Inspiratory lung volume derivative (direct calculation) ==
  v : Inport
  Enable : EnablePort
  Constant3 : Constant  Value=0
  Derivative : Derivative
  Max : MinMax  Function=max  Inputs=2
  dv+ : Outport
  wires:
  Constant3/1 -> Max/2
  v/1 -> Derivative/1
  Max/1 -> dv+/1  "dv+"
  Derivative/1 -> Max/1

== system ards_model/main-model/Lung volume model/Inspiratory lung volume derivative (fourier approximation) ==
  dVA : Inport
  omega*t : Inport  Port=2
  Enable : EnablePort
  Add2 : Sum
  Gain : Gain  Gain=pi
  Half-wave rectifier : Subsystem
  zero-prevention threshold : Constant  Value=0.01
  dv+ : Outport
  wires:
  omega*t/1 -> Half-wave rectifier/2(2pift)
  zero-prevention threshold/1 -> Add2/2
  Half-wave rectifier/1(out) -> Gain/1
  Add2/1 -> dv+/1  "dv+"
  Gain/1 -> Add2/1
  dVA/1 -> Half-wave rectifier/1((d)VA)

== system ards_model/main-model/Predicted Body Weight/IfThenElse ==
  if : Inport  OutDataTypeStr=boolean
  then : Inport  Port=2
  else : Inport  Port=3
  Merge : Merge
  NOT : Logic  Operator=NOT  IconShape=distinctive  AllPortsSameDT=off  OutDataTypeStr=boolean
  Subsystem1 : Subsystem
  Subsystem2 : Subsystem
  out : Outport
  wires:
  then/1 -> Subsystem1/1(in)
  Subsystem2/1(out) -> Merge/2
  if/1 -> NOT/1, Subsystem1/Enable
  else/1 -> Subsystem2/1(in)
  Subsystem1/1(out) -> Merge/1
  NOT/1 -> Subsystem2/Enable
  Merge/1 -> out/1

== system ards_model/main-model/cvs integrator/Subsystem ==
  In1 : Inport
  dxcvs : Inport  Port=2
  Bus Creator1 : BusCreator  Inputs=10  OutDataTypeStr=Bus: CardioVascularStateDerivative
      settings: InheritFromInputs=off
  Bus to Vector : BusToVector
  Demux1 : Demux  Outputs=10
  Product : Product
  dxcvs1 : Outport
  wires:
  Demux1/6 -> Bus Creator1/6
  Demux1/8 -> Bus Creator1/8
  Demux1/7 -> Bus Creator1/7
  Demux1/5 -> Bus Creator1/5
  Product/1 -> Demux1/1
  Bus to Vector/1 -> Product/2
  Demux1/4 -> Bus Creator1/4
  Demux1/9 -> Bus Creator1/9
  Demux1/10 -> Bus Creator1/10
  Demux1/1 -> Bus Creator1/1
  Demux1/2 -> Bus Creator1/2
  Demux1/3 -> Bus Creator1/3
  Bus Creator1/1 -> dxcvs1/1  "dxcvs"
  In1/1 -> Product/1  "a"
  dxcvs/1 -> Bus to Vector/1  "dxcvs"

== system ards_model/main-model/cvs integrator/Subsystem3 ==
  In1 : Inport  OutDataTypeStr=Bus: CardioVascularStateDerivative
  Enable : EnablePort
  Out1 : Outport  OutDataTypeStr=Bus: CardioVascularStateDerivative
  wires:
  In1/1 -> Out1/1

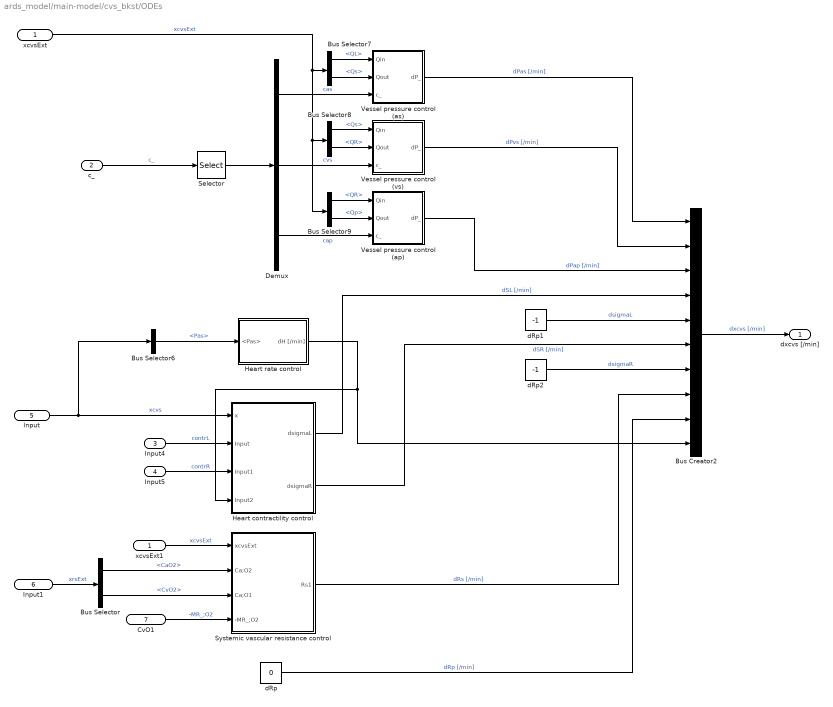
== system ards_model/main-model/cvs_bkst/ODEs ==
  xcvsExt : Inport  OutDataTypeStr=Bus: CardioVascularStateExtended
  c_ : Inport  Port=2  Unit=L/mmHg
  Input4 : Inport  Port=3  OutDataTypeStr=double  PortDimensions=3
  Input5 : Inport  Port=4  OutDataTypeStr=double  PortDimensions=3
  Input : Inport  Port=5  OutDataTypeStr=Bus: CardioVascularState
  Input1 : Inport  Port=6  OutDataTypeStr=Bus: RespiratoryStateExtended
  CvO1 : Inport  Port=7  Unit=L/min
  Bus Creator2 : BusCreator  Inputs=10  OutDataTypeStr=Bus: CardioVascularStateDerivative
  Bus Selector : BusSelector  OutputSignals=CaO2,CvO2
  Bus Selector6 : BusSelector  OutputSignals=Pas
  Bus Selector7 : BusSelector  OutputSignals=QL,Qs
  Bus Selector8 : BusSelector  OutputSignals=Qs,QR
  Bus Selector9 : BusSelector  OutputSignals=QR,Qp
  Demux : Demux  Outputs=3
  Heart contractility control : Subsystem
  Heart rate control : Subsystem
  Selector : Selector  InputPortWidth=4  IndexOptions=Index vector (dialog)  Indices=[1 2 3]  OutputSizes=1
  Systemic vascular resistance control : Subsystem
  Vessel pressure control (ap) : Subsystem
  Vessel pressure control (as) : Subsystem
  Vessel pressure control (vs) : Subsystem
  dRp : Constant  Value=0
  dRp1 : Constant  Value=-1
  dRp2 : Constant  Value=-1
  xcvsExt1 : InportShadow  OutDataTypeStr=Bus: CardioVascularStateExtended
  dxcvs [/min] : Outport  OutDataTypeStr=Bus: CardioVascularStateDerivative
  wires:
  Vessel pressure control (ap)/1(dP_) -> Bus Creator2/3  "dPap [/min]"
  Bus Selector8/1 -> Vessel pressure control (vs)/1(Qin)  "<Qs>"
  Vessel pressure control (vs)/1(dP_) -> Bus Creator2/2  "dPvs [/min]"
  CvO1/1 -> Systemic vascular resistance control/4(-MR_;O2)  "-MR_;O2"
  Demux/2 -> Vessel pressure control (vs)/3(c_)  "cvs"
  Bus Selector9/1 -> Vessel pressure control (ap)/1(Qin)  "<QR>"
  c_/1 -> Selector/1  "c_"
  Heart contractility control/1(dsigmaL) -> Bus Creator2/4  "dSL [/min]"
  Vessel pressure control (as)/1(dP_) -> Bus Creator2/1  "dPas [/min]"
  Demux/1 -> Vessel pressure control (as)/3(c_)  "cas"
  Systemic vascular resistance control/1(Rs1) -> Bus Creator2/8  "dRs [/min]"
  dRp/1 -> Bus Creator2/9  "dRp [/min]"
  xcvsExt/1 -> Bus Selector9/1, Bus Selector8/1, Bus Selector7/1  "xcvsExt"
  dRp2/1 -> Bus Creator2/7  "dsigmaR"
  xcvsExt1/1 -> Systemic vascular resistance control/1(xcvsExt)  "xcvsExt"
  Input/1 -> Heart contractility control/1(x), Bus Selector6/1  "xcvs"
  Input4/1 -> Heart contractility control/2(Input)  "contrL"
  Heart contractility control/2(dsigmaR) -> Bus Creator2/6  "dSR [/min]"
  dRp1/1 -> Bus Creator2/5  "dsigmaL"
  Input5/1 -> Heart contractility control/3(Input1)  "contrR"
  Bus Selector9/2 -> Vessel pressure control (ap)/2(Qout)  "<Qp>"
  Demux/3 -> Vessel pressure control (ap)/3(c_)  "cap"
  Selector/1 -> Demux/1
  Bus Creator2/1 -> dxcvs [/min]/1  "dxcvs [/min]"
  Bus Selector7/2 -> Vessel pressure control (as)/2(Qout)  "<Qs>"
  Bus Selector7/1 -> Vessel pressure control (as)/1(Qin)  "<QL>"
  Bus Selector/1 -> Systemic vascular resistance control/2(Ca;O2)  "<CaO2>"
  Input1/1 -> Bus Selector/1  "xrsExt"
  Bus Selector8/2 -> Vessel pressure control (vs)/2(Qout)  "<QR>"
  Bus Selector/2 -> Systemic vascular resistance control/3(Ca;O1)  "<CvO2>"
  Heart rate control/1(dH [/min]) -> Heart contractility control/4(Input2), Bus Creator2/10
  Bus Selector6/1 -> Heart rate control/1(<Pas>)  "<Pas>"

== system ards_model/main-model/cvs_bkst/Subsystem ==
  In1 : Inport
  Out1 : Outport
  wires:
  In1/1 -> Out1/1

== system ards_model/main-model/rs integrator/Subsystem ==
  In1 : Inport
  dxcvs : Inport  Port=2
  Bus Creator1 : BusCreator  Inputs=6  OutDataTypeStr=Bus: RespiratoryStateDerivative
      settings: InheritFromInputs=off
  Bus to Vector : BusToVector
  Demux1 : Demux  Outputs=6
  Product : Product
  dxcvs1 : Outport
  wires:
  Product/1 -> Demux1/1
  Bus to Vector/1 -> Product/2
  Bus Creator1/1 -> dxcvs1/1  "dxrs"
  In1/1 -> Product/1  "a"
  dxcvs/1 -> Bus to Vector/1  "dxrs"
  Demux1/1 -> Bus Creator1/1
  Demux1/2 -> Bus Creator1/2
  Demux1/3 -> Bus Creator1/3
  Demux1/4 -> Bus Creator1/4
  Demux1/5 -> Bus Creator1/5
  Demux1/6 -> Bus Creator1/6

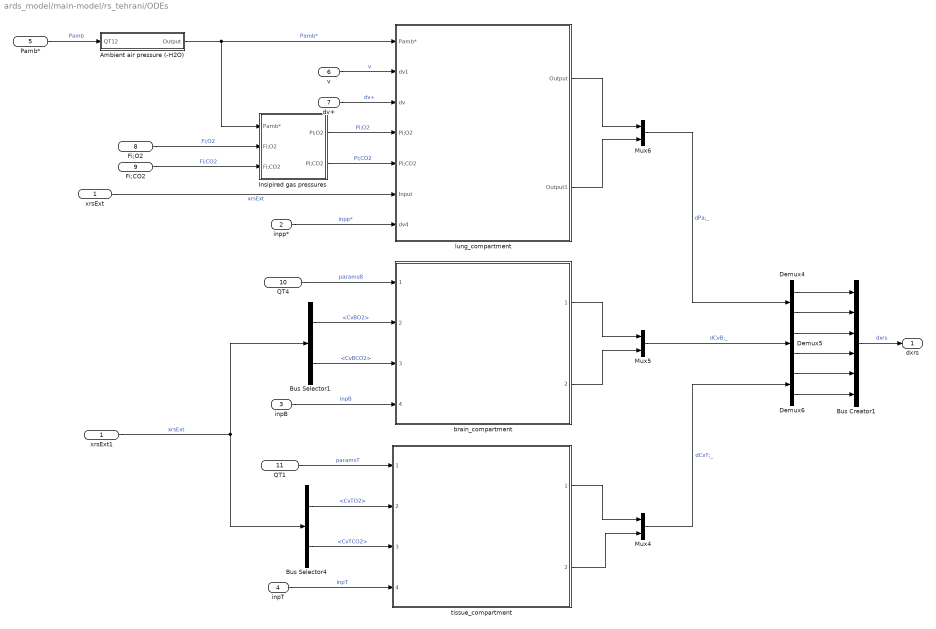
== system ards_model/main-model/rs_tehrani/ODEs ==
  xrsExt : Inport  OutDataTypeStr=Bus: RespiratoryStateExtended
  inpp* : Inport  Port=2  OutDataTypeStr=Bus: BloodGasFlow
  inpB : Inport  Port=3  OutDataTypeStr=Bus: BloodGasFlow
  inpT : Inport  Port=4  OutDataTypeStr=Bus: BloodGasFlow
  Pamb* : Inport  Port=5  Unit=mmHg
  v : Inport  Port=6  Unit=L
  dv+ : Inport  Port=7  Unit=L/s
  Fi;O2 : Inport  Port=8  Unit=1
  Fi;CO2 : Inport  Port=9  Unit=1
  QT4 : Inport  Port=10  PortDimensions=3
  QT1 : Inport  Port=11  PortDimensions=3
  Ambient air pressure (-H2O) : Subsystem  TreatAsAtomicUnit=on
  Bus Creator1 : BusCreator  Inputs=6  OutDataTypeStr=Bus: RespiratoryStateDerivative
      settings: InheritFromInputs=off
  Bus Selector1 : BusSelector  OutputSignals=CvBO2,CvBCO2
  Bus Selector4 : BusSelector  OutputSignals=CvTO2,CvTCO2
  Demux4 : Demux  Outputs=2
  Demux5 : Demux  Outputs=2
  Demux6 : Demux  Outputs=2
  Insipired gas pressures : Subsystem  TreatAsAtomicUnit=on
  Mux4 : Mux  Inputs=2
  Mux5 : Mux  Inputs=2
  Mux6 : Mux  Inputs=2
  brain_compartment : Subsystem  ReferencedSubsystem=tehrani_tissue_compartment_v2
  lung_compartment : Subsystem
  tissue_compartment : Subsystem  ReferencedSubsystem=tehrani_tissue_compartment_v2
  xrsExt1 : InportShadow  OutDataTypeStr=Bus: RespiratoryStateExtended
  dxrs : Outport  OutDataTypeStr=Bus: RespiratoryStateDerivative
  wires:
  xrsExt1/1 -> Bus Selector4/1, Bus Selector1/1  "xrsExt"
  Fi;O2/1 -> Insipired gas pressures/2(Fi;O2)  "Fi;O2"
  Bus Selector1/2 -> brain_compartment/3  "<CvBCO2>"
  Ambient air pressure (-H2O)/1(Output) -> lung_compartment/1(Pamb*), Insipired gas pressures/1(Pamb*)  "Pamb*"
  Demux4/2 -> Bus Creator1/2
  Fi;CO2/1 -> Insipired gas pressures/3(Fi;CO2)  "Fi;CO2"
  Bus Selector1/1 -> brain_compartment/2  "<CvBO2>"
  Demux4/1 -> Bus Creator1/1
  Pamb*/1 -> Ambient air pressure (-H2O)/1(QT12)  "Pamb"
  tissue_compartment/2 -> Mux4/2
  Demux5/1 -> Bus Creator1/3
  tissue_compartment/1 -> Mux4/1
  Demux6/1 -> Bus Creator1/5
  Demux5/2 -> Bus Creator1/4
  Demux6/2 -> Bus Creator1/6
  Mux5/1 -> Demux5/1  "dCvB;_"
  brain_compartment/1 -> Mux5/1
  inpT/1 -> tissue_compartment/4  "inpT"
  Mux6/1 -> Demux4/1  "dPa;_"
  brain_compartment/2 -> Mux5/2
  Bus Selector4/1 -> tissue_compartment/2  "<CvTO2>"
  Mux4/1 -> Demux6/1  "dCvT;_"
  Bus Selector4/2 -> tissue_compartment/3  "<CvTCO2>"
  inpB/1 -> brain_compartment/4  "inpB"
  Bus Creator1/1 -> dxrs/1  "dxrs"
  v/1 -> lung_compartment/2(dv1)  "v"
  dv+/1 -> lung_compartment/3(dv)  "dv+"
  Insipired gas pressures/1(Pi;O2) -> lung_compartment/4(Pi;O2)  "Pi;O2"
  Insipired gas pressures/2(Pi;CO2) -> lung_compartment/5(Pi;CO2)  "Pi;CO2"
  xrsExt/1 -> lung_compartment/6(Input)  "xrsExt"
  inpp*/1 -> lung_compartment/7(dv4)  "inpp*"
  lung_compartment/1(Output) -> Mux6/1
  lung_compartment/2(Output1) -> Mux6/2
  QT4/1 -> brain_compartment/1  "paramsB"
  QT1/1 -> tissue_compartment/1  "paramsT"

== system ards_model/ards_classification/Berlin definition/ards_level/ards_level_string ==
  In1 : Inport
  In2 : Inport  Port=2
  In3 : Inport  Port=3
  In4 : Inport  Port=4
  Merge : Merge  Inputs=4
  String Constant : StringConstant  String="\"severe\""
  String Constant1 : StringConstant  String="\"moderate\""
  String Constant2 : StringConstant  String="\"mild\""
  String Constant3 : StringConstant  String="\"no\""
  Subsystem : Subsystem
  Subsystem1 : Subsystem
  Subsystem2 : Subsystem
  Subsystem3 : Subsystem
  ards_level : Outport
  wires:
  Subsystem1/1(out) -> Merge/2
  Merge/1 -> ards_level/1  "ards_level"
  Subsystem/1(out) -> Merge/1
  In1/1 -> Subsystem/Enable  "severe"
  Subsystem3/1(out) -> Merge/4
  Subsystem2/1(out) -> Merge/3
  String Constant/1 -> Subsystem/1(in)
  String Constant1/1 -> Subsystem1/1(in)
  In2/1 -> Subsystem1/Enable  "moderate"
  In3/1 -> Subsystem2/Enable  "mild"
  In4/1 -> Subsystem3/Enable  "no"
  String Constant2/1 -> Subsystem2/1(in)
  String Constant3/1 -> Subsystem3/1(in)

== system ards_model/ards_classification/Berlin definition/ards_level/ards_level_switch ==
  horowitz : Inport  Unit=mmHg
  horowitz1 : Inport  Port=2  Unit=1
  Pamb1 : Inport  Port=3  Unit=m
  Pamb : Inport  Port=4  Unit=mmHg
  AND : Logic  IconShape=distinctive  AllPortsSameDT=off  OutDataTypeStr=boolean
  AND1 : Logic  IconShape=distinctive  AllPortsSameDT=off  OutDataTypeStr=boolean
  LessThan1 : RelationalOperator  Operator=<=  OutDataTypeStr=boolean  RndMeth=Simplest
  LessThan2 : RelationalOperator  Operator=<=  OutDataTypeStr=boolean  RndMeth=Simplest
  LessThan3 : RelationalOperator  Operator=<=  OutDataTypeStr=boolean  RndMeth=Simplest
  NOT : Logic  Operator=NOT  IconShape=distinctive  AllPortsSameDT=off  OutDataTypeStr=boolean
  NOT1 : Logic  Operator=NOT  IconShape=distinctive  AllPortsSameDT=off  OutDataTypeStr=boolean
  NOT2 : Logic  Operator=NOT  IconShape=distinctive  AllPortsSameDT=off  OutDataTypeStr=boolean
  correction : Subsystem
  mild : Constant  Value=300
  moderate : Constant  Value=200
  severe : Constant  Value=100
  issevere : Outport
  ismoderate : Outport  Port=2
  ismild : Outport  Port=3
  isno : Outport  Port=4
  wires:
  severe/1 -> LessThan1/2
  mild/1 -> LessThan2/2
  LessThan1/1 -> issevere/1, NOT/1  "severe"
  NOT1/1 -> AND1/1
  LessThan2/1 -> AND1/2, NOT2/1
  LessThan3/1 -> AND/2, NOT1/1
  AND1/1 -> ismild/1  "mild"
  NOT/1 -> AND/1
  moderate/1 -> LessThan3/2
  NOT2/1 -> isno/1  "no"
  AND/1 -> ismoderate/1  "moderate"
  correction/1(horowitz*) -> LessThan2/1, LessThan3/1, LessThan1/1
  Pamb1/1 -> correction/3(altitude)  "altitude"
  horowitz1/1 -> correction/2(Fi;O2)  "Fi;O2"
  Pamb/1 -> correction/4(Pamb)  "Pamb"
  horowitz/1 -> correction/1(horowitz)  "horowitz"

== system ards_model/ards_classification/eGFR_CKD-EPI/alpha/Enabled Subsystem ==
  In1 : Inport
  Enable : EnablePort
  Out1 : Outport
  wires:
  In1/1 -> Out1/1

== system ards_model/ards_classification/eGFR_CKD-EPI/alpha/Enabled Subsystem1 ==
  In1 : Inport
  Enable : EnablePort
  Out1 : Outport
  wires:
  In1/1 -> Out1/1

== system ards_model/ards_classification/eGFR_CKD-EPI/kappa/Enabled Subsystem ==
  In1 : Inport
  Enable : EnablePort
  Out1 : Outport
  wires:
  In1/1 -> Out1/1

== system ards_model/ards_classification/eGFR_CKD-EPI/kappa/Enabled Subsystem1 ==
  In1 : Inport
  Enable : EnablePort
  Out1 : Outport
  wires:
  In1/1 -> Out1/1

== system ards_model/ards_classification/eGFR_CKD-EPI/sex factor/Enabled Subsystem ==
  In1 : Inport
  Enable : EnablePort
  Out1 : Outport
  wires:
  In1/1 -> Out1/1

== system ards_model/ards_classification/eGFR_CKD-EPI/sex factor/Enabled Subsystem1 ==
  In1 : Inport
  Enable : EnablePort
  Out1 : Outport
  wires:
  In1/1 -> Out1/1

== system ards_model/ards_classification/eGFR_CKD-EPI/skin color factor/Enabled Subsystem ==
  In1 : Inport
  Enable : EnablePort
  Out1 : Outport
  wires:
  In1/1 -> Out1/1

== system ards_model/ards_classification/eGFR_CKD-EPI/skin color factor/Enabled Subsystem1 ==
  In1 : Inport
  Enable : EnablePort
  Out1 : Outport
  wires:
  In1/1 -> Out1/1

== system ards_model/ards_classification/logFon_score/Compliance/Blood volume estimate ==
  note: Total blood volume by body surface
      | Source: [BKST] ch 1.6.1a [Altman and Dittmer, 1971, p. 376 ff.]
      | Vtot = 3.290 s - 1.229
  surface : Inport  Unit=m^2
  Add4 : Sum  Inputs=+-
  Constant1 : Constant  Value=3.290
  Constant2 : Constant  Value=1.229
  Product2 : Product
  Vtot : Outport  Unit=L
  wires:
  Constant2/1 -> Add4/2
  Product2/1 -> Add4/1
  Constant1/1 -> Product2/2
  Add4/1 -> Vtot/1  "Vtot"
  surface/1 -> Product2/1  "surface"

== system ards_model/ards_classification/logFon_score/Compliance/Body surface estimate ==
  note: s = 0.007184 w^0.425 h^0.725
      |
      | source: CVRS ch 1.6.1 [Du Bois’ formula (Keidl, 1985, p. 377)]
      | WolframAlpha
  height : Inport  Unit=m
  Weight : Inport  Port=2  Unit=kg
  Constant1 : Constant  Value=0.007184
  Constant2 : Constant  Value=0.725
  Constant3 : Constant  Value=0.425
  Gain : Gain  Gain=100
  Power : Math  Operator=pow  SaturateOnIntegerOverflow=on
  Power1 : Math  Operator=pow  SaturateOnIntegerOverflow=on
  Product2 : Product  Inputs=***
  surface : Outport  Unit=m^2
  wires:
  Power1/1 -> Product2/2
  Constant2/1 -> Power/2
  Constant1/1 -> Product2/3
  Product2/1 -> surface/1  "surface"
  Constant3/1 -> Power1/2
  Power/1 -> Product2/1
  Weight/1 -> Power1/1  "weight"
  height/1 -> Gain/1  "height"
  Gain/1 -> Power/1  "height [cm]"

== system ards_model/ards_classification/logFon_score/Compliance/Initial blood volume distribution ==
  note: Initial four-compartment distribution of total blood volume
      | source: [BKST] ch 1.6.1b
  Vtot : Inport  Unit=L
  Constant1 : Constant  Value=0.514
  Constant2 : Constant  Value=0.212
  Constant3 : Constant  Value=0.107
  Constant4 : Constant  Value=0.167
  Product{2..5} (4 alike) : Product
  V_as : Outport  Unit=L
  V_as1 : Outport  Port=2  Unit=L
  V_as2 : Outport  Port=3  Unit=L
  V_as3 : Outport  Port=4  Unit=L
  wires:
  Constant1/1 -> Product3/2
  Constant3/1 -> Product4/2
  Product2/1 -> V_as/1  "Vas;0"
  Vtot/1 -> Product2/1, Product3/1, Product4/1, Product5/1
  Constant4/1 -> Product5/2
  Constant2/1 -> Product2/2
  Product3/1 -> V_as1/1  "Vvs;0"
  Product4/1 -> V_as2/1  "Vap;0"
  Product5/1 -> V_as3/1  "Vvp;0"

== system ards_model/ards_classification/logFon_score/Compliance/Vessel compliances ==
  In5 : Inport  Unit=L
  In6 : Inport  Port=2  Unit=L
  In7 : Inport  Port=3  Unit=L
  In8 : Inport  Port=4  Unit=L
  Constant : Constant  Value=P_default
  Demux : Demux
  Vessel compliance (ap) : Subsystem  ReferencedSubsystem=vessel_compliance
  Vessel compliance (as) : Subsystem  ReferencedSubsystem=vessel_compliance
  Vessel compliance (vp) : Subsystem  ReferencedSubsystem=vessel_compliance
  Vessel compliance (vs) : Subsystem  ReferencedSubsystem=vessel_compliance
  cas : Outport  Unit=L/mmHg
  cvs : Outport  Port=2  Unit=L/mmHg
  cap : Outport  Port=3  Unit=L/mmHg
  cvp : Outport  Port=4  Unit=L/mmHg
  wires:
  Demux/3 -> Vessel compliance (ap)/2  "Pap;default"
  In5/1 -> Vessel compliance (as)/1  "Vas;0"
  In7/1 -> Vessel compliance (ap)/1  "Vap;0"
  Demux/2 -> Vessel compliance (vs)/2  "Pvs;default"
  Vessel compliance (vp)/1 -> cvp/1  "cvp"
  Demux/4 -> Vessel compliance (vp)/2  "Pvp;default"
  In6/1 -> Vessel compliance (vs)/1  "Vvs;0"
  Demux/1 -> Vessel compliance (as)/2  "Pas;default"
  Vessel compliance (ap)/1 -> cap/1  "cap"
  In8/1 -> Vessel compliance (vp)/1  "Vvp;0"
  Vessel compliance (as)/1 -> cas/1  "cas"
  Vessel compliance (vs)/1 -> cvs/1  "cvs"
  Constant/1 -> Demux/1  "P_;default"
